simulink subsystem "Calculate_Frenet_and_Paths"  (R2022b)
settings: Solver=VariableStepAuto  StartTime=0.0  StopTime=10.0  RelTol=1e-3
settings Model: Creator=User  LastModifiedBy=User

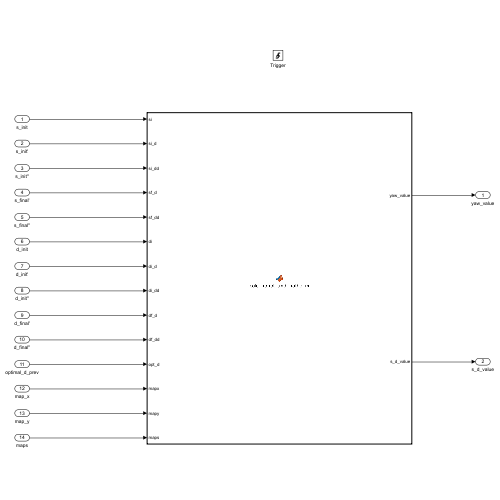
[thumbnail: Simulink's stored preview of the top-level diagram]
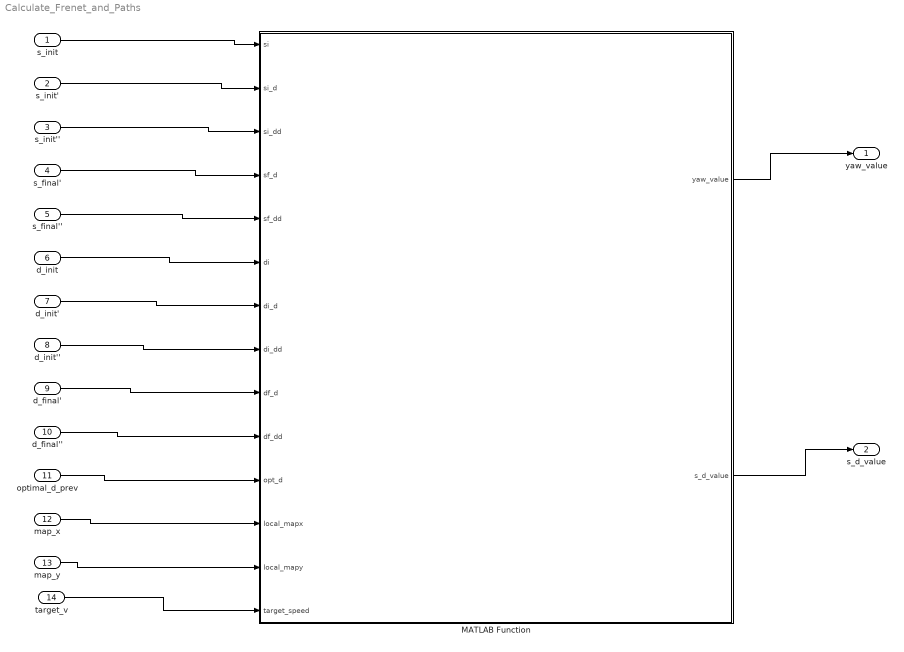
== system Calculate_Frenet_and_Paths ==
  s_init : Inport
  s_init' : Inport  Port=2
  s_init'' : Inport  Port=3
  s_final' : Inport  Port=4
  s_final'' : Inport  Port=5
  d_init : Inport  Port=6
  d_init' : Inport  Port=7
  d_init'' : Inport  Port=8
  d_final' : Inport  Port=9
  d_final'' : Inport  Port=10
  optimal_d_prev : Inport  Port=11
  map_x : Inport  Port=12
  map_y : Inport  Port=13
  target_v : Inport  Port=14
  MATLAB Function : MATLAB Function  TreatAsAtomicUnit=on
  yaw_value : Outport
  s_d_value : Outport  Port=2
  wires:
  s_init/1 -> MATLAB Function/1(si)
  s_init'/1 -> MATLAB Function/2(si_d)
  s_init''/1 -> MATLAB Function/3(si_dd)
  s_final'/1 -> MATLAB Function/4(sf_d)
  s_final''/1 -> MATLAB Function/5(sf_dd)
  d_init/1 -> MATLAB Function/6(di)
  d_init'/1 -> MATLAB Function/7(di_d)
  d_init''/1 -> MATLAB Function/8(di_dd)
  d_final'/1 -> MATLAB Function/9(df_d)
  d_final''/1 -> MATLAB Function/10(df_dd)
  optimal_d_prev/1 -> MATLAB Function/11(opt_d)
  map_x/1 -> MATLAB Function/12(local_mapx)
  map_y/1 -> MATLAB Function/13(local_mapy)
  MATLAB Function/1(yaw_value) -> yaw_value/1
  MATLAB Function/2(s_d_value) -> s_d_value/1
  target_v/1 -> MATLAB Function/14(target_speed)

== matlab function Calculate_Frenet_and_Paths/MATLAB Function ==
  data: si input; yaw_value output; si_d input; si_dd input; sf_d input; sf_dd input; di input; di_d input; di_dd input; df_d input; df_dd input; opt_d input; local_mapx input; local_mapy input; s_d_value output; target_speed input
function [yaw_value, s_d_value] = calculate_frenet_and_local_paths_m(si, si_d, si_dd, sf_d, sf_dd, di, di_d, di_dd, df_d, df_dd, opt_d, local_mapx, local_mapy, target_speed)
    [yaw_value, s_d_value] = calculate_frenet_and_local_paths(si, si_d, si_dd, sf_d, sf_dd, di, di_d, di_dd, df_d, df_dd, opt_d, local_mapx, local_mapy, target_speed);
    
end
